simulink model "6DoF_V11_2024a_AirspeedHold"  (R2024a)
settings: Solver=ode45  StartTime=0.0  StopTime=300  FixedStep=.01  MaxStep=.004  RelTol=1e-5  EnableMultiTasking=on
values from neighbouring files (symbols this model uses):
  ac = [0 0 0]    [Geom_6dof_V4_WITH_MAP.m]
  b = 33.4    [Geom_6dof_V4_WITH_MAP.m]
  Bank_rate = zeros(1,length(points))    [Geom_6dof_V4_WITH_MAP.m]
  cbar = 5.7    [Geom_6dof_V4_WITH_MAP.m]
  cda2 = 0.33    [Geom_6dof_V4_WITH_MAP.m]
  cdo = 0.05    [Geom_6dof_V4_WITH_MAP.m]
  cg = [0 0 0]    [Geom_6dof_V4_WITH_MAP.m]
  cla = 4.44    [Geom_6dof_V4_WITH_MAP.m]
  cladot = 0    [Geom_6dof_V4_WITH_MAP.m]
  clb = -0.074    [Geom_6dof_V4_WITH_MAP.m]
  clda = -0.134    [Geom_6dof_V4_WITH_MAP.m]
  clde = 0.355    [Geom_6dof_V4_WITH_MAP.m]
  cldr = 0.107    [Geom_6dof_V4_WITH_MAP.m]
  clo = 0.41    [Geom_6dof_V4_WITH_MAP.m]
  clp = -0.410    (= -0.41)    [Geom_6dof_V4_WITH_MAP.m]
  clq = 3.8    [Geom_6dof_V4_WITH_MAP.m]
  clr = 0.107    [Geom_6dof_V4_WITH_MAP.m]
  cma = -0.683    [Geom_6dof_V4_WITH_MAP.m]
  cmadot = -4.36    [Geom_6dof_V4_WITH_MAP.m]
  cmde = -0.923    [Geom_6dof_V4_WITH_MAP.m]
  cmq = -9.96    [Geom_6dof_V4_WITH_MAP.m]
  cnb = 0.071    [Geom_6dof_V4_WITH_MAP.m]
  cnda = -0.0035    [Geom_6dof_V4_WITH_MAP.m]
  cndr = -0.072    [Geom_6dof_V4_WITH_MAP.m]
  cnp = -0.0575    [Geom_6dof_V4_WITH_MAP.m]
  cnr = -0.125    [Geom_6dof_V4_WITH_MAP.m]
  cyb = -0.564    [Geom_6dof_V4_WITH_MAP.m]
  cydr = 0.157    [Geom_6dof_V4_WITH_MAP.m]
  eng = [0 0 0]    [Geom_6dof_V4_WITH_MAP.m]
  finlat = 37.8044    [Geom_6dof_V4_WITH_MAP.m]
  finlong = -122.2712    [Geom_6dof_V4_WITH_MAP.m]
  initalt = 5000    [Geom_6dof_V4_WITH_MAP.m]
  initbank = 0    [Geom_6dof_V4_WITH_MAP.m]
  initeast = 0    [Geom_6dof_V4_WITH_MAP.m]
  inithead = 0    [Geom_6dof_V4_WITH_MAP.m]
  initlat = 37.7749    [Geom_6dof_V4_WITH_MAP.m]
  initlong = -122.4194    [Geom_6dof_V4_WITH_MAP.m]
  initnorth = 0    [Geom_6dof_V4_WITH_MAP.m]
  initp = 0    [Geom_6dof_V4_WITH_MAP.m]
  initpitch = initw/initu    (= -0.0287187462721)    [Geom_6dof_V4_WITH_MAP.m]
  initq = 0    [Geom_6dof_V4_WITH_MAP.m]
  initr = 0    [Geom_6dof_V4_WITH_MAP.m]
  initu = 226.333    [Geom_6dof_V4_WITH_MAP.m]
  initv = 0    [Geom_6dof_V4_WITH_MAP.m]
  initw = -6.5    [Geom_6dof_V4_WITH_MAP.m]
  jx = 1048    [Geom_6dof_V4_WITH_MAP.m]
  jxz = 0    [Geom_6dof_V4_WITH_MAP.m]
  jy = 3000    [Geom_6dof_V4_WITH_MAP.m]
  jz = 3500    [Geom_6dof_V4_WITH_MAP.m]
  points = (-180:180)*(pi()/180)    [Geom_6dof_V4_WITH_MAP.m]
  RB_Bank = zeros(1,length(points))    [Geom_6dof_V4_WITH_MAP.m]
  sw = 184    [Geom_6dof_V4_WITH_MAP.m]
  weight = 2750    [Geom_6dof_V4_WITH_MAP.m]
  WP1 = [10000 10000 5000]    [Geom_6dof_V4_WITH_MAP.m]
  WP2 = [-10000 0 5500]    [Geom_6dof_V4_WITH_MAP.m]
  WP3 = [0 -10000 4500]    [Geom_6dof_V4_WITH_MAP.m]
libraries: slpidlib x14, simulink_extras x5, dspswit3 x1
(part 3 of 3)

== system 6DoF_V11_2024a_AirspeedHold/Aircraft_Dynamics/Aerodynamics/Aero Forces and Moments/Aerodynamic Forces ==
  CD : Inport
  CY : Inport  Port=2
  CL : Inport  Port=3
  Wind Para : Inport  Port=4
  dyn(q) : Inport  Port=5
  Body to Wind : Subsystem
  Demux : Demux  Outputs=3
      settings: DisplayOption=none
  Gain : Gain  Gain=-1  SaturateOnIntegerOverflow=on  OutDataTypeStr=Inherit: Same as input  ParamDataTypeStr=Inherit: Same as input
  Gain1 : Gain  Gain=-1  SaturateOnIntegerOverflow=on  OutDataTypeStr=Inherit: Same as input  ParamDataTypeStr=Inherit: Same as input
  Gain2 : Gain  Gain=sw  SaturateOnIntegerOverflow=on  OutDataTypeStr=Inherit: Same as input  ParamDataTypeStr=Inherit: Same as input
  Math Function : Math  Operator=transpose  SignedPower=on
  Mux : Mux  Inputs=3
  Product : Product  SaturateOnIntegerOverflow=on  OutDataTypeStr=Inherit: Same as first input
  Product1 : Product  Multiplication=Matrix(*)  SaturateOnIntegerOverflow=on  OutDataTypeStr=Inherit: Same as first input
  Terminator : Terminator
  FaeroBody : Outport
  wires:
  Gain/1 -> Mux/1
  Gain1/1 -> Mux/3
  Mux/1 -> Product/1
  Gain2/1 -> Product/2
  CD/1 -> Gain/1
  CY/1 -> Mux/2
  CL/1 -> Gain1/1
  dyn(q)/1 -> Gain2/1
  Wind Para/1 -> Demux/1
  Demux/1 -> Terminator/1
  Body to Wind/1(Smatrix) -> Math Function/1
  Math Function/1 -> Product1/1
  Product/1 -> Product1/2
  Product1/1 -> FaeroBody/1
  Demux/2 -> Body to Wind/1(Alpha)
  Demux/3 -> Body to Wind/2(Beta)

== system 6DoF_V11_2024a_AirspeedHold/Aircraft_Dynamics/Aerodynamics/Aero Forces and Moments/Aerodynamic Moments ==
  dyn(q) : Inport
  Croll : Inport  Port=2
  CM : Inport  Port=3
  CN : Inport  Port=4
  Mux : Mux  Inputs=2
  Mux1 : Mux  Inputs=2
  Mux2 : Mux  Inputs=2
  Mux3 : Mux  Inputs=3
  Pitch : Fcn  Expr=u[1] * sw * cbar * u[2]
  Roll : Fcn  Expr=u[1] * sw * b * u[2]
  Yaw : Fcn  Expr=u[1] * sw * b * u[2]
  Maero : Outport
  wires:
  Mux/1 -> Roll/1
  Mux1/1 -> Pitch/1
  Mux2/1 -> Yaw/1
  Pitch/1 -> Mux3/2
  Roll/1 -> Mux3/1
  Yaw/1 -> Mux3/3
  dyn(q)/1 -> Mux/1, Mux1/1, Mux2/1
  Croll/1 -> Mux/2
  CM/1 -> Mux1/2
  CN/1 -> Mux2/2
  Mux3/1 -> Maero/1

== system 6DoF_V11_2024a_AirspeedHold/Aircraft_Dynamics/Aerodynamics/CD/Get Alpha ==
  windPar : Inport
  "   " : Terminator
  "   1" : Terminator
  Demux : Demux  Outputs=3
      settings: DisplayOption=none
  Alpha : Outport
  wires:
  Demux/1 -> "   1"/1
  Demux/3 -> "   "/1
  windPar/1 -> Demux/1
  Demux/2 -> Alpha/1

== system 6DoF_V11_2024a_AirspeedHold/Aircraft_Dynamics/Equations of motion numerical integration /Kinematic Equiations/2pi Bound ==
  In : Inport
  2pi : Constant  Value=2*pi
  Math Function : Math  Operator=mod  SignedPower=on
  Out : Outport
  wires:
  Math Function/1 -> Out/1
  2pi/1 -> Math Function/2
  In/1 -> Math Function/1

== system 6DoF_V11_2024a_AirspeedHold/Aircraft_Dynamics/Equations of motion numerical integration /Kinematic Equiations/pi Bound ==
  In : Inport
  2pi : Constant  Value=2*pi
  Math Function : Math  Operator=mod  SignedPower=on
  Sum1 : Sum  Inputs=|+-  InputSameDT=on  SaturateOnIntegerOverflow=on  OutDataTypeStr=Inherit: Same as first input
  Sum2 : Sum  Inputs=|++  InputSameDT=on  SaturateOnIntegerOverflow=on  OutDataTypeStr=Inherit: Same as first input
  pi : Constant  Value=pi
  Out : Outport
  wires:
  Sum1/1 -> Out/1
  pi/1 -> Sum1/2, Sum2/2
  Sum2/1 -> Math Function/1
  In/1 -> Sum2/1
  2pi/1 -> Math Function/2
  Math Function/1 -> Sum1/1

== system 6DoF_V11_2024a_AirspeedHold/Aircraft_Dynamics/Equations of motion numerical integration /Kinematic Equiations/pi Bound1 ==
  In : Inport
  2pi : Constant  Value=2*pi
  Math Function : Math  Operator=mod  SignedPower=on
  Sum1 : Sum  Inputs=|+-  InputSameDT=on  SaturateOnIntegerOverflow=on  OutDataTypeStr=Inherit: Same as first input
  Sum2 : Sum  Inputs=|++  InputSameDT=on  SaturateOnIntegerOverflow=on  OutDataTypeStr=Inherit: Same as first input
  pi : Constant  Value=pi
  Out : Outport
  wires:
  Sum1/1 -> Out/1
  pi/1 -> Sum1/2, Sum2/2
  Sum2/1 -> Math Function/1
  In/1 -> Sum2/1
  2pi/1 -> Math Function/2
  Math Function/1 -> Sum1/1

== system 6DoF_V11_2024a_AirspeedHold/Aircraft_Dynamics/Equations of motion numerical integration /Moment Equations/Inertia Coefs ==
  note: Jx,Jy,Jz,Jxz
  note: Inertia Coefficeents
      | Page 80 Stevens and Lewis
  Inertia : Inport
  Mux : Mux  Inputs=9
  c1 : Fcn  Expr=((u[2]-u[3])*u[3] - u[4]^2)/(u[1]*u[3]-u[4]^2)
  c2 : Fcn  Expr=((u[1]-u[2]+u[3])*u[4])/(u[1]*u[3]-u[4]^2)
  c3 : Fcn  Expr=u[3]/(u[1]*u[3]-u[4]^2)
  c4 : Fcn  Expr=u[4]/(u[1]*u[3]-u[4]^2)
  c5 : Fcn  Expr=(u[3]-u[1])/u[2]
  c6 : Fcn  Expr=u[4]/u[2]
  c7 : Fcn  Expr=1/u[2]
  c8 : Fcn  Expr=(u[1]*(u[1]-u[2])+u[4]^2)/(u[1]*u[3]-u[4]^2)
  c9 : Fcn  Expr=u[1]/(u[1]*u[3]-u[4]^2)
  Iner Coef : Outport
  wires:
  Inertia/1 -> c1/1, c2/1, c3/1, c4/1, c5/1, c6/1, c7/1, c9/1, c8/1
  c1/1 -> Mux/1
  c2/1 -> Mux/2
  c3/1 -> Mux/3
  c4/1 -> Mux/4
  c5/1 -> Mux/5
  c6/1 -> Mux/6
  c7/1 -> Mux/7
  c8/1 -> Mux/8
  c9/1 -> Mux/9
  Mux/1 -> Iner Coef/1

== system 6DoF_V11_2024a_AirspeedHold/Aircraft_Dynamics/Aerodynamics/Aero Forces and Moments/Aerodynamic Forces/Body to Wind ==
  note: This transforms any arbitrary vector from body axis to wind axis.
      | Page 63  Stevens and Lewis
  Alpha : Inport
  Beta : Inport  Port=2
  -ca sb : Fcn  Expr=-1 * cos(u[1]) * sin(u[2])
  -sa : Fcn  Expr=-1 * sin(u[1])
  -sa sb : Fcn  Expr="-1 * sin(u[1])  * sin(u[2])"
  Fcn8 : Fcn  Expr=cos(u[1])
  Matrix Concatenation : Concatenate  NumInputs=3  Mode=Multidimensional array
  Matrix Concatenation1 : Concatenate  NumInputs=3  Mode=Multidimensional array
  Matrix Concatenation2 : Concatenate  NumInputs=3  Mode=Multidimensional array  ConcatenateDimension=2
  Matrix Concatenation3 : Concatenate  NumInputs=3  Mode=Multidimensional array
  Mux1 : Mux  Inputs=2
  ca cb : Fcn  Expr="cos(u[1]) *  cos(u[2])"
  cb : Fcn  Expr=cos(u[2])
  sa cb : Fcn  Expr=sin(u[1]) * cos(u[2])
  sb : Fcn  Expr=sin(u[2])
  zero : Fcn  Expr=u[1] * 0
  Smatrix : Outport
  wires:
  Matrix Concatenation/1 -> Matrix Concatenation2/1
  Matrix Concatenation1/1 -> Matrix Concatenation2/2
  Matrix Concatenation3/1 -> Matrix Concatenation2/3
  -ca sb/1 -> Matrix Concatenation/2
  ca cb/1 -> Matrix Concatenation/1
  -sa/1 -> Matrix Concatenation/3
  zero/1 -> Matrix Concatenation1/3
  sb/1 -> Matrix Concatenation1/1
  cb/1 -> Matrix Concatenation1/2
  sa cb/1 -> Matrix Concatenation3/1
  -sa sb/1 -> Matrix Concatenation3/2
  Fcn8/1 -> Matrix Concatenation3/3
  Mux1/1 -> ca cb/1, -ca sb/1, -sa/1, sb/1, cb/1, zero/1, sa cb/1, -sa sb/1, Fcn8/1
  Alpha/1 -> Mux1/1
  Beta/1 -> Mux1/2
  Matrix Concatenation2/1 -> Smatrix/1
